simulink model "CSTR"  (R2020a)
settings: Solver=VariableStepAuto  StartTime=0.0  StopTime=10.0  RelTol=1e-3
settings Model: Creator=mac  LastModifiedBy=mac

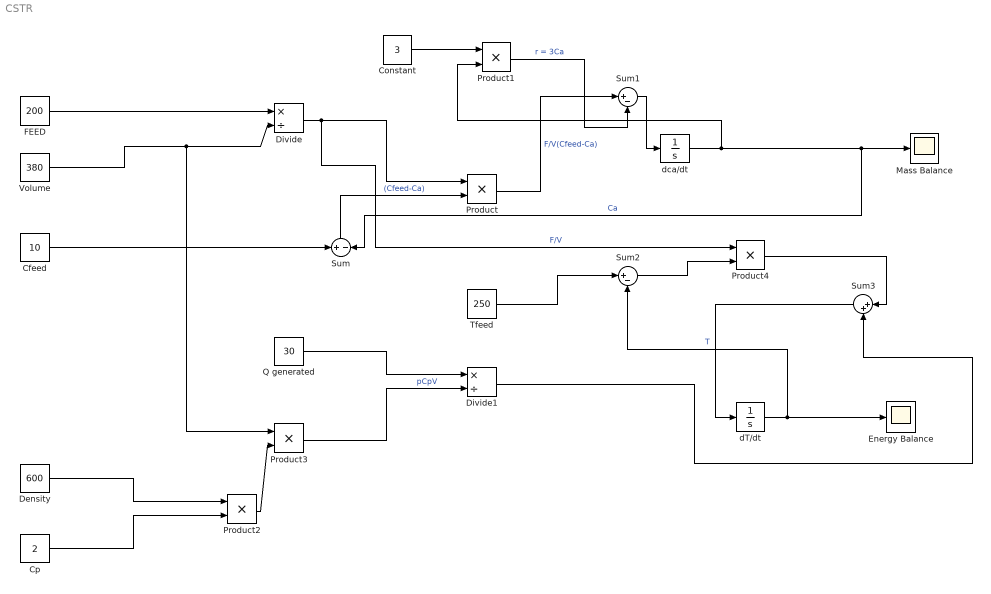
== system CSTR ==
  "Cfeed " : Constant  Value=10
  Constant : Constant  Value=3
  Cp : Constant  Value=2
  "Density " : Constant  Value=600
  Divide : Product  Inputs=*/
  Divide1 : Product  Inputs=*/
  "Energy Balance " : Scope
  FEED : Constant  Value=200
  "Mass Balance " : Scope
  Product{,1..4} (5 alike) : Product
  "Q generated " : Constant  Value=30
  Sum : Sum  Inputs=+-
  Sum1 : Sum  Inputs=|+-
  Sum2 : Sum  Inputs=|+-
  Sum3 : Sum  Inputs=|++
  Tfeed : Constant  Value=250
  "Volume " : Constant  Value=380
  dT/dt : Integrator
  dca/dt : Integrator  InitialCondition=100
  wires:
  FEED/1 -> Divide/1
  "Volume "/1 -> Product3/1, Divide/2
  "Cfeed "/1 -> Sum/1
  Divide/1 -> Product4/1, Product/1  "F/V"
  Sum/1 -> Product/2  "(Cfeed-Ca)"
  Sum1/1 -> dca/dt/1
  Constant/1 -> Product1/1
  dca/dt/1 -> Product1/2, Sum/2, "Mass Balance "/1  "Ca"
  Product1/1 -> Sum1/2  "r = 3Ca"
  Product/1 -> Sum1/1  "F/V(Cfeed-Ca)"
  "Density "/1 -> Product2/1
  Cp/1 -> Product2/2
  Product2/1 -> Product3/2
  "Q generated "/1 -> Divide1/1
  Product3/1 -> Divide1/2  "pCpV"
  dT/dt/1 -> "Energy Balance "/1, Sum2/2  "T"
  Tfeed/1 -> Sum2/1
  Sum2/1 -> Product4/2
  Product4/1 -> Sum3/1
  Divide1/1 -> Sum3/2
  Sum3/1 -> dT/dt/1
